simulink model "LQR_balance_control_2020"  (R2023b)
settings: Solver=ode1  StartTime=0.0  StopTime=inf  FixedStep=0.002  RelTol=1e-3  EnableMultiTasking=on
PostLoadFcn:
  | qc_set_target_type(getConfigSet(bdroot, 'QUARC Default Target Configuration'));
undefined symbols (not defined in the file or in its folder): HIL, K, Lp, qc_get_step_size
libraries: quarc_library x11, simulink_extras x2, simulink x1
settings Model: SimulationMode=external  ExtModeTrigDuration=5000  Creator=pmartin  LastModifiedBy=sameb
settings SolverCC: AlgebraicLoopSolver=TrustRegion  PositivePriorityOrder=on  AutoInsertRateTranBlk=on
settings DataIOCC: LimitDataPoints=on  SaveFormat=Array  SignalLoggingSaveFormat=ModelDataLogs  ReturnWorkspaceOutputs=off
settings OptimizationCC: ExpressionDepthLimit=2147483647  InitFltsAndDblsToZero=on
settings DebuggingCC: SaveWithParameterizedLinksMsg=none  UnderspecifiedInitializationDetection=Classic  MergeDetectMultiDrivingBlocksExec=none  SolverPrmCheckMsg=warning  MultiTaskDSMMsg=warning  MultiTaskCondExecSysMsg=none  FcnCallInpInsideContextMsg=warning  UnconnectedInputMsg=warning  UnconnectedOutputMsg=warning  UnconnectedLineMsg=warning  StateNameClashWarn=warning  SFUnexpectedBacktrackingDiag=warning  SFNoUnconditionalDefaultTransitionDiag=warning  SFExecutionAtInitializationDiag=none  ArithmeticOperatorsInVariantConditions=warning
settings HardwareCC: ProdBitPerPointer=32  ProdBitPerSizeT=32  ProdBitPerPtrDiffT=32  ProdLargestAtomicFloat=None  ProdIntDivRoundTo=Undefined  ProdEndianess=Unspecified  ProdWordSize=32  ProdHWDeviceType=32-bit Generic
settings ModelReferenceCC: EnableRefExpFcnMdlSchedulingChecks=on  PropagateSignalLabelsOutOfModel=off
settings SFSimCC: SimUseLocalCustomCode=off  CustomCodeUndefinedFunction=UseInterfaceOnly
settings RTWCC: Description=QUARC Win64 Target  SystemTargetFile=quarc_win64.tlc  TemplateMakefile=quarc_default_tmf  RTWUseLocalCustomCode=off  DLArmComputeVersion=19.05
settings CodeAppCC: StateflowObjectComments=on
settings STFCustomTargetCC: TargetPreCompLibLocation=C:\PROGRA~3\QUARC\lib\2020b\win64\release  TargetLangStandard=C89/C90 (ANSI)  ConcurrentExecutionCompliant=on  GRTInterface=on  SystemTargetFile=quarc_win64.tlc
settings GRTTargetCC: TargetPreCompLibLocation=C:\PROGRA~3\QUARC\lib\2020b\win64\release  TargetLangStandard=C89/C90 (ANSI)  ParMdlRefBuildCompliant=off  CompOptLevelCompliant=off  CombineOutputUpdateFcns=off  MatFileLogging=off  CPPClassGenCompliant=off  GRTInterface=on  UseToolchainInfoCompliant=off  ExtMode=on  ExtModeMexFile=quarc_comm
settings ConfigComp: CovMetricSettings=dw  CovSaveCumulativeToWorkspaceVar=on  CovSaveSingleToWorkspaceVar=on  CovExternalEMLEnable=off

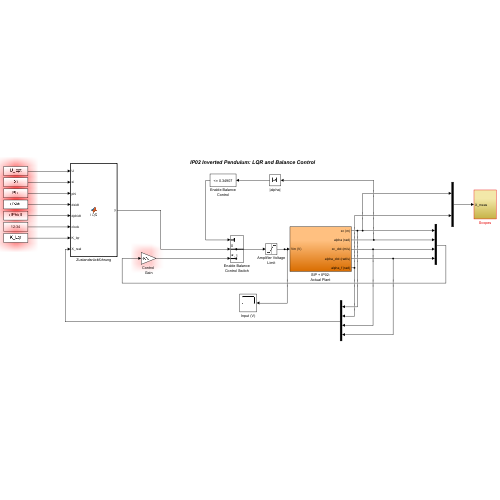
[thumbnail: Simulink's stored preview of the top-level diagram]
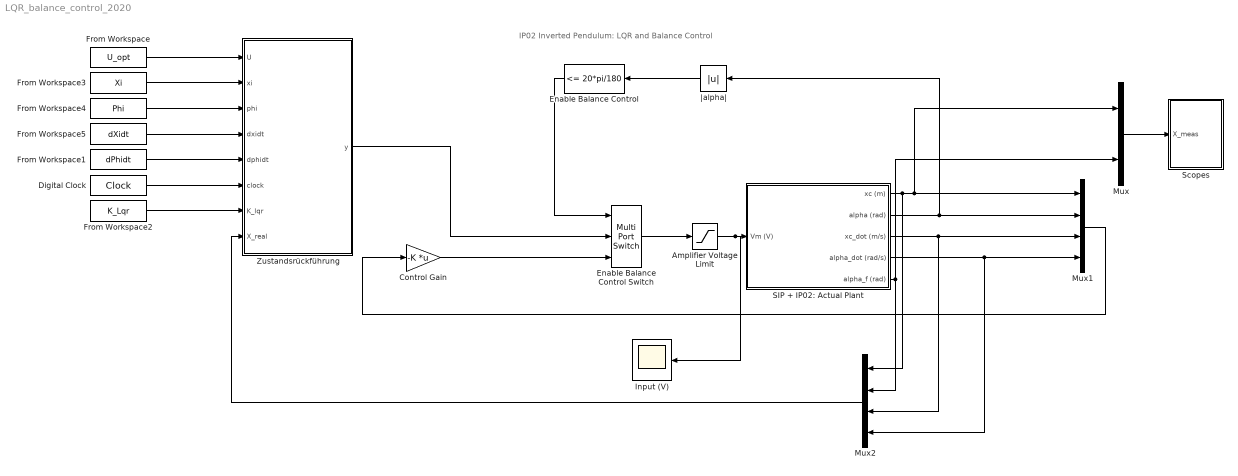
== system LQR_balance_control_2020 ==
  note: IP02 Inverted Pendulum: LQR and Balance Control
  Amplifier Voltage Limit : Saturate  UpperLimit=10  LowerLimit=-10
  Control Gain : Gain  Gain=-K  Multiplication=Matrix(K*u)
  Digital Clock : DigitalClock  SampleTime=0.01
  Enable Balance Control : simulink/Logic and Bit Operations/Compare To Constant  relop=<=  const=20*pi/180  OutDataTypeStr=uint8  ZeroCross=off
  Enable Balance Control Switch : MultiPortSwitch  DataPortOrder=Zero-based contiguous  Inputs=2  zeroidx=on  SaturateOnIntegerOverflow=off  InputSameDT=off
  From Workspace : FromWorkspace  VariableName=U_opt
  From Workspace1 : FromWorkspace  VariableName=dPhidt
  From Workspace2 : FromWorkspace  VariableName=K_Lqr
  From Workspace3 : FromWorkspace  VariableName=Xi
  From Workspace4 : FromWorkspace  VariableName=Phi
  From Workspace5 : FromWorkspace  VariableName=dXidt
  Input (V) : Scope
  Mux : Mux  Inputs=2
  Mux1 : Mux
  Mux2 : Mux
  SIP + IP02: Actual Plant : Subsystem
  Scopes : Subsystem
  Zustandsrückführung : MATLAB Function  TreatAsAtomicUnit=on
  |alpha| : Abs  SaturateOnIntegerOverflow=off
  wires:
  Amplifier Voltage Limit/1 -> Input (V)/1, SIP + IP02: Actual Plant/1(Vm (V))
  Mux1/1 -> Control Gain/1
  Enable Balance Control/1 -> Enable Balance Control Switch/1
  Control Gain/1 -> Enable Balance Control Switch/3
  SIP + IP02: Actual Plant/1(xc (m)) -> Mux2/1, Mux/1, Mux1/1
  |alpha|/1 -> Enable Balance Control/1
  SIP + IP02: Actual Plant/2(alpha (rad)) -> |alpha|/1, Mux1/2
  Zustandsrückführung/1(y) -> Enable Balance Control Switch/2
  From Workspace/1 -> Zustandsrückführung/1(U)
  From Workspace3/1 -> Zustandsrückführung/2(xi)
  From Workspace4/1 -> Zustandsrückführung/3(phi)
  From Workspace5/1 -> Zustandsrückführung/4(dxidt)
  From Workspace1/1 -> Zustandsrückführung/5(dphidt)
  Digital Clock/1 -> Zustandsrückführung/6(clock)
  SIP + IP02: Actual Plant/4(alpha_dot (rad/s)) -> Mux2/4, Mux1/4
  SIP + IP02: Actual Plant/3(xc_dot (m/s)) -> Mux2/3, Mux1/3
  Mux2/1 -> Zustandsrückführung/8(X_real)
  Mux/1 -> Scopes/1(X_meas)
  SIP + IP02: Actual Plant/5(alpha_f (rad)) -> Mux2/2, Mux/2
  From Workspace2/1 -> Zustandsrückführung/7(K_lqr)
  Enable Balance Control Switch/1 -> Amplifier Voltage Limit/1

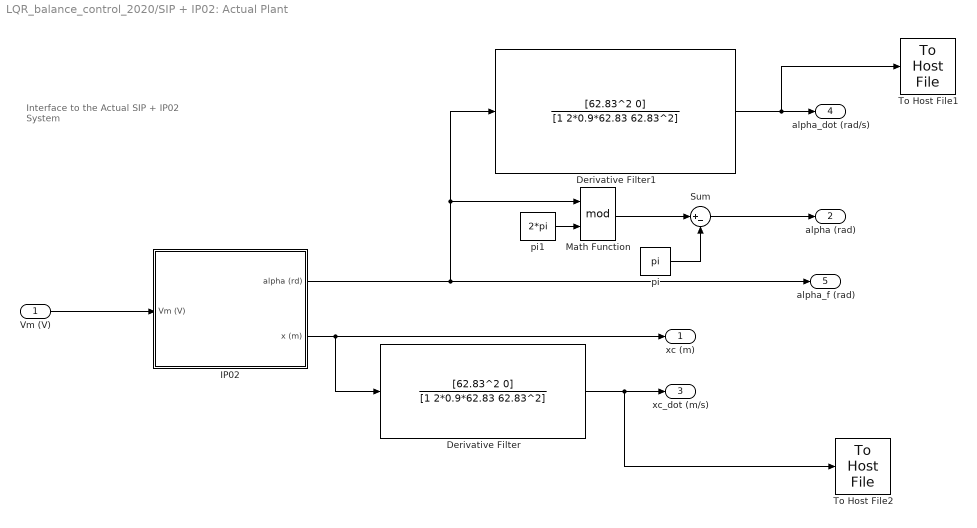
== system LQR_balance_control_2020/SIP + IP02: Actual Plant ==
  note: Interface to the Actual
      | SIP + IP02 System
  Vm (V) : Inport
  Derivative Filter : TransferFcn  Numerator=[62.83^2 0]  Denominator=[1 2*0.9*62.83 62.83^2]
  Derivative Filter1 : TransferFcn  Numerator=[62.83^2 0]  Denominator=[1 2*0.9*62.83 62.83^2]
  "IP02 " : Subsystem
  Math Function : Math  Operator=mod  SignedPower=on
  Sum : Sum  Inputs=|+-  InputSameDT=on  SaturateOnIntegerOverflow=on  OutDataTypeStr=Inherit: Same as first input
  To Host File1 : quarc_library/Sinks/To Host/To Host File  file_name=alphadt_meas.mat  variable_name=alphadt_meas  decimation=1  sample_time=0.01  file_format=MAT-file v.4  options=No header or footer  append=off  final_file_name=alphadt_meas.mat  bitrate=2000000
  To Host File2 : quarc_library/Sinks/To Host/To Host File  file_name=xdt_meas.mat  variable_name=xdt_meas  decimation=1  sample_time=0.01  file_format=MAT-file v.4  options=No header or footer  append=off  final_file_name=xdt_meas.mat  bitrate=2000000
  pi : Constant  Value=pi
  pi1 : Constant  Value=2*pi
  xc (m) : Outport  InitialOutput=0
  alpha (rad) : Outport  Port=2  InitialOutput=0
  xc_dot (m/s) : Outport  Port=3  InitialOutput=0
  alpha_dot (rad/s) : Outport  Port=4  InitialOutput=0
  alpha_f (rad) : Outport  Port=5  InitialOutput=0
  wires:
  "IP02 "/2(x (m)) -> xc (m)/1, Derivative Filter/1
  Derivative Filter1/1 -> To Host File1/1, alpha_dot (rad/s)/1
  pi1/1 -> Math Function/2
  pi/1 -> Sum/2
  Sum/1 -> alpha (rad)/1
  Math Function/1 -> Sum/1
  Vm (V)/1 -> "IP02 "/1(Vm (V))
  "IP02 "/1(alpha (rd)) -> Math Function/1, Derivative Filter1/1, alpha_f (rad)/1
  Derivative Filter/1 -> To Host File2/1, xc_dot (m/s)/1

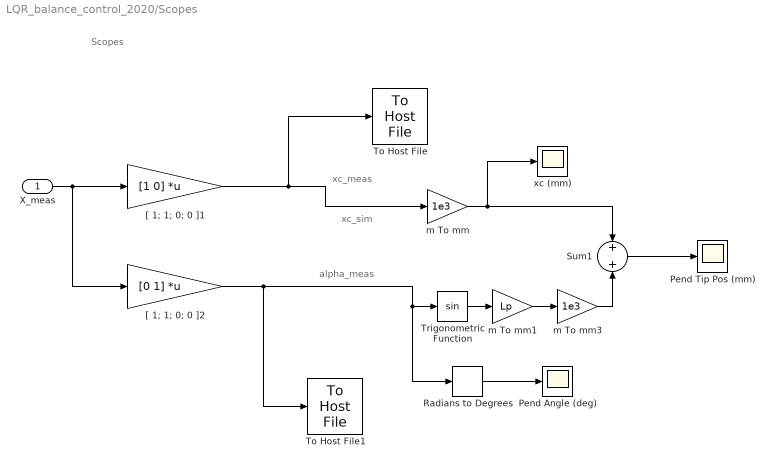
== system LQR_balance_control_2020/Scopes ==
  note: xc_meas
  note: alpha_meas
  note: xc_sim
  note: Scopes
  X_meas : Inport
  Pend Angle (deg) : Scope
  Pend Tip Pos (mm) : Scope
  Radians to Degrees : simulink_extras/Transformations/Radians to Degrees
  Sum1 : Sum  Inputs=+|+  InputSameDT=on  SaturateOnIntegerOverflow=on  OutDataTypeStr=Inherit: Same as first input
  To Host File : quarc_library/Sinks/To Host/To Host File  file_name=x_meas.mat  variable_name=x_meas  decimation=1  sample_time=0.01  file_format=MAT-file v.4  options=No header or footer  append=off  final_file_name=x_meas.mat  bitrate=2000000
  To Host File1 : quarc_library/Sinks/To Host/To Host File  file_name=alpha_meas.mat  variable_name=alpha_meas  decimation=1  sample_time=0.01  file_format=MAT-file v.4  options=No header or footer  append=off  final_file_name=alpha_meas.mat  bitrate=2000000
  Trigonometric Function : Trigonometry
  "[ 1; 1; 0; 0 ]1" : Gain  Gain=[1 0]  Multiplication=Matrix(K*u)  SaturateOnIntegerOverflow=on  OutDataTypeStr=Inherit: Same as input  ParamDataTypeStr=Inherit: Same as input
  "[ 1; 1; 0; 0 ]2" : Gain  Gain=[0 1]  Multiplication=Matrix(K*u)  SaturateOnIntegerOverflow=on  OutDataTypeStr=Inherit: Same as input  ParamDataTypeStr=Inherit: Same as input
  m To mm : Gain  Gain=1e3  SaturateOnIntegerOverflow=on  OutDataTypeStr=Inherit: Same as input  ParamDataTypeStr=Inherit: Same as input
  m To mm1 : Gain  Gain=Lp  SaturateOnIntegerOverflow=on  OutDataTypeStr=Inherit: Same as input  ParamDataTypeStr=Inherit: Same as input
  m To mm3 : Gain  Gain=1e3  SaturateOnIntegerOverflow=on  OutDataTypeStr=Inherit: Same as input  ParamDataTypeStr=Inherit: Same as input
  xc (mm) : Scope
  wires:
  m To mm/1 -> Sum1/1, xc (mm)/1
  X_meas/1 -> "[ 1; 1; 0; 0 ]1"/1, "[ 1; 1; 0; 0 ]2"/1
  m To mm1/1 -> m To mm3/1
  Trigonometric Function/1 -> m To mm1/1
  m To mm3/1 -> Sum1/2
  Sum1/1 -> Pend Tip Pos (mm)/1
  Radians to Degrees/1 -> Pend Angle (deg)/1
  "[ 1; 1; 0; 0 ]1"/1 -> To Host File/1, m To mm/1
  "[ 1; 1; 0; 0 ]2"/1 -> To Host File1/1, Trigonometric Function/1, Radians to Degrees/1

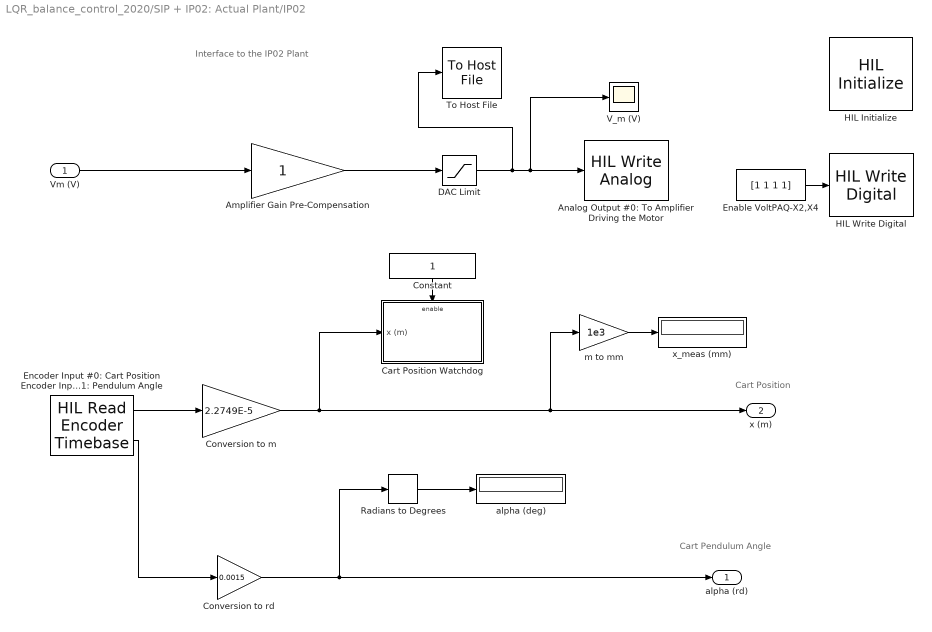
== system LQR_balance_control_2020/SIP + IP02: Actual Plant/IP02  ==
  note: Cart Pendulum Angle
  note: Cart Position
  note: Interface to the IP02 Plant
  Vm (V) : Inport
  Amplifier Gain Pre-Compensation : Gain  SaturateOnIntegerOverflow=on  OutDataTypeStr=Inherit: Same as input  ParamDataTypeStr=Inherit: Same as input
  Analog Output #0: To Amplifier Driving the Motor : quarc_library/Data Acquisition/Generic/Immediate I//O/HIL Write Analog  Tag=unassigned  object_name=HIL-1  channels=0  sample_time=-1  active=on  vector_input=on
  Cart Position Watchdog : Subsystem  TreatAsAtomicUnit=on
  Constant : Constant
  Conversion to m : Gain  Gain=2.2749E-5  SaturateOnIntegerOverflow=on  OutDataTypeStr=Inherit: Same as input  ParamDataTypeStr=Inherit: Same as input
  Conversion to rd : Gain  Gain=0.0015  SaturateOnIntegerOverflow=on  OutDataTypeStr=Inherit: Same as input  ParamDataTypeStr=Inherit: Same as input
  DAC Limit : Saturate  UpperLimit=10  LowerLimit=-10
  Enable VoltPAQ-X2,X4 : Constant  Value=[1 1 1 1]
  Encoder Input #0: Cart Position Encoder Input #1: Pendulum Angle : quarc_library/Data Acquisition/Generic/Timebases/HIL Read Encoder Timebase  Tag=unassigned  object_name=HIL-1  clock=0  channels=[0 1]  active=on  vector_output=off  data_type_mode=Inherit via back propagation  data_type=double  overflow_mode=Error on overflow  samples_in_buffer=max(ceil(1/qc_get_step_size), 1)
  HIL Initialize : quarc_library/Data Acquisition/Generic/Configuration/HIL Initialize  object_name=HIL-1  board_type=q2_usb  board_number=0  board_options=d0=digital;d1=digital;led=auto;update_rate=normal  exclusive=off  active=off  hardware_clocks=[0:2]  clock_modes=[]  initial_clock_frequencies=[]  set_clock_params_at_start=off  set_clock_params_at_switch_in=off  set_clock_frequencies_at_start=off  set_clock_frequencies_at_switch_in=off  analog_input_channels=[0:1]  analog_input_configurations=[]  analog_input_maximums=10  analog_input_minimums=-10  set_analog_input_params_at_start=on  set_analog_input_params_at_switch_in=off  analog_output_channels=[0:1]  analog_output_maximums=10  analog_output_minimums=-10  initial_analog_outputs=[0]  final_analog_outputs=[0]  watchdog_analog_outputs=0  set_analog_output_params_at_start=on  set_analog_output_params_at_switch_in=off  set_analog_outputs_at_start=on  set_analog_outputs_at_switch_in=off  set_analog_outputs_at_terminate=on  set_analog_outputs_at_switch_out=off  set_analog_outputs_on_watchdog=off  digital_input_channels=[]  digital_output_channels=[0:7]  digital_output_configuration=[]  initial_digital_outputs=[0]  final_digital_outputs=[0]  watchdog_digital_outputs=[0]  set_digital_output_params_at_start=off  set_digital_output_params_at_switch_in=off  set_digital_outputs_at_start=on  set_digital_outputs_at_switch_in=off  set_digital_outputs_at_terminate=on  set_digital_outputs_at_switch_out=off  set_digital_outputs_on_watchdog=off  encoder_channels=[0:1]  quadrature=[4]  encoder_filter_frequency=[]  initial_encoder_counts=[0]  set_encoder_params_at_start=on  set_encoder_params_at_switch_in=off  set_encoder_counts_at_start=on  set_encoder_counts_at_switch_in=off  pwm_channels=[]  pwm_modes=[0]  pwm_frequency=1/0.020  pwm_configuration=[]  pwm_alignment=[]  pwm_polarity=[]  pwm_leading_deadband=[]  pwm_trailing_deadband=[]  initial_pwm_outputs=[0]  final_pwm_outputs=[0]  watchdog_pwm_outputs=[0]  set_pwm_params_at_start=on  set_pwm_params_at_switch_in=off  set_pwm_outputs_at_start=on  set_pwm_outputs_at_switch_in=off  set_pwm_outputs_at_terminate=on  set_pwm_outputs_at_switch_out=off  set_pwm_outputs_on_watchdog=off  other_output_channels=[]  initial_other_outputs=[]  final_other_outputs=[]  watchdog_other_outputs=[]  set_other_outputs_at_start=off  set_other_outputs_at_switch_in=off  set_other_outputs_at_terminate=off  set_other_outputs_at_switch_out=off  set_other_outputs_on_watchdog=off
  HIL Write Digital : quarc_library/Data Acquisition/Generic/Immediate I//O/HIL Write Digital  object_name=HIL-1  channels=[0:3]  sample_time=-1  active=off  vector_input=on
  Radians to Degrees : simulink_extras/Transformations/Radians to Degrees
  To Host File : quarc_library/Sinks/To Host/To Host File  file_name=input.mat  variable_name=input  decimation=1  sample_time=0.01  file_format=MAT-file v.4  options=No header or footer  append=off  final_file_name=input.mat  bitrate=2000000
  V_m (V) : Scope
  alpha (deg) : Display
      settings: Decimation=100
  m to mm : Gain  Gain=1e3  SaturateOnIntegerOverflow=on  OutDataTypeStr=Inherit: Same as input  ParamDataTypeStr=Inherit: Same as input
  x_meas (mm) : Display
      settings: Decimation=100
  alpha (rd) : Outport  InitialOutput=0
  x (m) : Outport  Port=2  InitialOutput=0
  wires:
  Encoder Input #0: Cart Position Encoder Input #1: Pendulum Angle/1 -> Conversion to m/1
  Conversion to m/1 -> Cart Position Watchdog/1(x (m)), x (m)/1, m to mm/1
  Amplifier Gain Pre-Compensation/1 -> DAC Limit/1
  m to mm/1 -> x_meas (mm)/1
  Encoder Input #0: Cart Position Encoder Input #1: Pendulum Angle/2 -> Conversion to rd/1
  Radians to Degrees/1 -> alpha (deg)/1
  Conversion to rd/1 -> Radians to Degrees/1, alpha (rd)/1
  Constant/1 -> Cart Position Watchdog/Enable
  Vm (V)/1 -> Amplifier Gain Pre-Compensation/1
  Enable VoltPAQ-X2,X4/1 -> HIL Write Digital/1
  DAC Limit/1 -> To Host File/1, Analog Output #0: To Amplifier Driving the Motor/1, V_m (V)/1

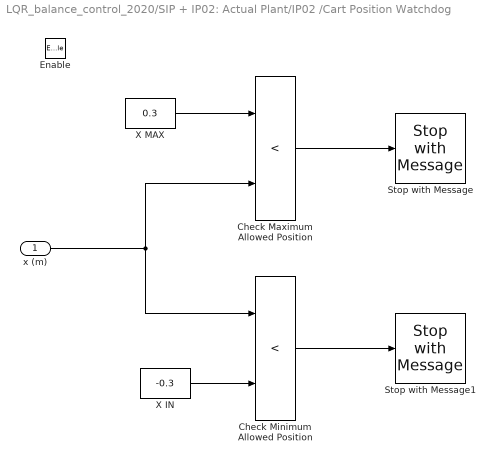
== system LQR_balance_control_2020/SIP + IP02: Actual Plant/IP02 /Cart Position Watchdog ==
  x (m) : Inport
  Enable : EnablePort
  Check Maximum Allowed Position : RelationalOperator  Operator=<
  Check Minimum Allowed Position : RelationalOperator  Operator=<
  Stop with Message : quarc_library/Sinks/Error Handling/Stop with Message  message_type=Fixed error message  message_icon=Error  message=Maximum Limit Reached.
  Stop with Message1 : quarc_library/Sinks/Error Handling/Stop with Message  message_type=Fixed error message  message_icon=Error  message=Minimum Limit Reached.
  X IN : Constant  Value=-0.3
  X MAX : Constant  Value=0.3
  wires:
  Check Maximum Allowed Position/1 -> Stop with Message/1
  x (m)/1 -> Check Minimum Allowed Position/1, Check Maximum Allowed Position/2
  X IN/1 -> Check Minimum Allowed Position/2
  Check Minimum Allowed Position/1 -> Stop with Message1/1
  X MAX/1 -> Check Maximum Allowed Position/1

== matlab function LQR_balance_control_2020/Zustandsrückführung ==
  data: U input; xi input; phi input; dxidt input; dphidt input; clock input; K_lqr input; X_real input; y output
function y = LQR(U,xi,phi,dxidt,dphidt,clock,K_lqr, X_real)
if (clock > 1.82) 
    y = 0;
%elseif (clock > 2.61 && clock < 3)
%    y = U;
else
    dx1= [1 0 0 0]*X_real-xi;
    dx2= [0 1 0 0]*X_real-phi;
    dx3= [0 0 1 0]*X_real-dxidt;
    dx4= [0 0 0 1]*X_real-dphidt;
    dx = [dx1;dx2;dx3;dx4];
    u=-K_lqr'*dx+U;
    y = u;
end
